simulink model "PID_nonlinear_improved_practical"  (R2022b)
settings: Solver=VariableStepAuto  StartTime=0.0  StopTime=20  RelTol=1e-3
values from neighbouring files (symbols this model uses):
  bias_acc = rand*0.05-0.025    [config.m]
  bias_gyro = rand*10-5    [config.m]
  f = 0.035    [config.m]
  g = 9.8    [config.m]
  Jx = 2*Mc*R^2/5 + 2*m*l^2    (= 0.0448)    [config.m]
  Jy = 2*Mc*R^2/5 + 2*m*l^2    (= 0.0448)    [config.m]
  Jz = 2*Mc*R^2/5 + 4*m*l^2    (= 0.0808)    [config.m]
  Kd_pitch = 15    [config.m]
  Kd_roll = 15    [config.m]
  Kd_yaw = 15    [config.m]
  Kd_z = 15    [config.m]
  Ki_pitch = 1    [config.m]
  Ki_roll = 1    [config.m]
  Ki_yaw = 1    [config.m]
  Ki_z = 10    [config.m]
  Kp_pitch = 80    [config.m]
  Kp_roll = 80    [config.m]
  Kp_yaw = 80    [config.m]
  Kp_z = 80    [config.m]
  M = Mc + 4*m    (= 3)    [config.m]
  S = 0.6231    [config.m]
  Wind_phi = 0    [config.m]
  Wind_theta = 0    [config.m]
  WorkTemperature = 30    [config.m]
libraries: simulink x2
settings Model: Creator=cxk  LastModifiedBy=cxk

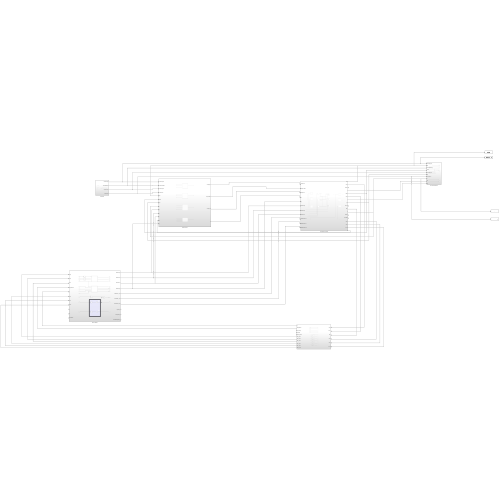
[thumbnail: Simulink's stored preview of the top-level diagram]
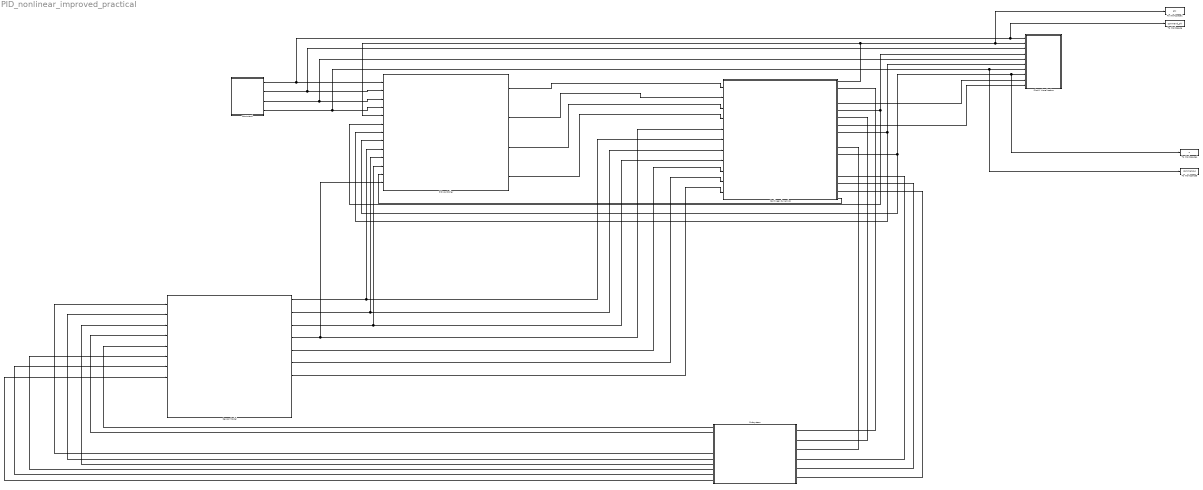
== system PID_nonlinear_improved_practical ==
  Command : Subsystem
  Nonlinear dynamics : Subsystem
  PID controller : Subsystem
  Plot & Visualization : Subsystem
  Sensor Model : Subsystem
  Subsystem : Subsystem
  To Workspace : ToWorkspace  VariableName=command_phi  SaveFormat=Timeseries  SampleTime=-1
  To Workspace1 : ToWorkspace  VariableName=phi  SaveFormat=Timeseries  SampleTime=-1
  To Workspace4 : ToWorkspace  VariableName=z  SaveFormat=Timeseries  SampleTime=-1
  To Workspace5 : ToWorkspace  VariableName=command_z  SaveFormat=Timeseries  SampleTime=-1
  wires:
  Nonlinear dynamics/8(psi) -> PID controller/7(psi), Plot & Visualization/6(psi)
  Nonlinear dynamics/5(theta) -> PID controller/6(theta), Plot & Visualization/4(theta)
  PID controller/4(F) -> Nonlinear dynamics/4(F)
  PID controller/1(Torque phi) -> Nonlinear dynamics/1(Torque Phi)
  PID controller/2(Torque theta) -> Nonlinear dynamics/2(Torque Theta)
  PID controller/3(Torque psi) -> Nonlinear dynamics/3(Torque Psi)
  Command/3(command psi) -> PID controller/3("command psi "), Plot & Visualization/5(command psi)
  Command/2(command theta) -> PID controller/2(command theta), Plot & Visualization/3(command theta)
  Nonlinear dynamics/4(x) -> Plot & Visualization/9(pn)
  Nonlinear dynamics/7(y) -> Plot & Visualization/10(pe)
  Subsystem/1(g) -> Sensor Model/5(g)
  Subsystem/2(temperature) -> Sensor Model/4(Temperature)
  Sensor Model/4(Measured g) -> Nonlinear dynamics/5(g), PID controller/13(g)
  Subsystem/6(dot p_real) -> Sensor Model/1(dot p)
  Subsystem/7(dot q_real) -> Sensor Model/2(dot q)
  Subsystem/8(dot r_real) -> Sensor Model/3(dot r)
  Subsystem/9(dot u_real) -> Sensor Model/6(dot u)
  Subsystem/10(dot v_real) -> Sensor Model/7(dot v)
  Subsystem/11(dot w_real) -> Sensor Model/8(dot w)
  Sensor Model/1(Measured p) -> Nonlinear dynamics/6(measured p), PID controller/9(p)
  Sensor Model/2(Measured q) -> Nonlinear dynamics/7(measured q), PID controller/10(q)
  Sensor Model/3(Measured r) -> Nonlinear dynamics/8(measured r), PID controller/11(r)
  Nonlinear dynamics/2(dot p) -> Subsystem/1(dot p)
  Nonlinear dynamics/6(dot q) -> Subsystem/2("dot q ")
  Nonlinear dynamics/10(dot r) -> Subsystem/3(dot r)
  Nonlinear dynamics/14(dot u) -> Subsystem/4(dot u)
  Nonlinear dynamics/15(dot v) -> Subsystem/5(dot v)
  Nonlinear dynamics/16(dot w) -> Subsystem/6(dot w)
  Sensor Model/5(Measured u_dot) -> Nonlinear dynamics/9(measured dot u)
  Sensor Model/6(Measured v_dot) -> Nonlinear dynamics/10(measured dot v)
  Sensor Model/7(Measured w_dot) -> Nonlinear dynamics/11(measured dot w)
  Nonlinear dynamics/17(w) -> PID controller/12(w)
  Nonlinear dynamics/11(z) -> PID controller/8(z), To Workspace4/1, Plot & Visualization/8(z)
  Nonlinear dynamics/1(Phi) -> To Workspace1/1, Plot & Visualization/2(phi), PID controller/5(phi)
  Command/4(command z) -> To Workspace5/1, Plot & Visualization/7(command z), PID controller/4(command z)
  Command/1(command phi) -> PID controller/1(command phi), To Workspace/1, Plot & Visualization/1(command phi)

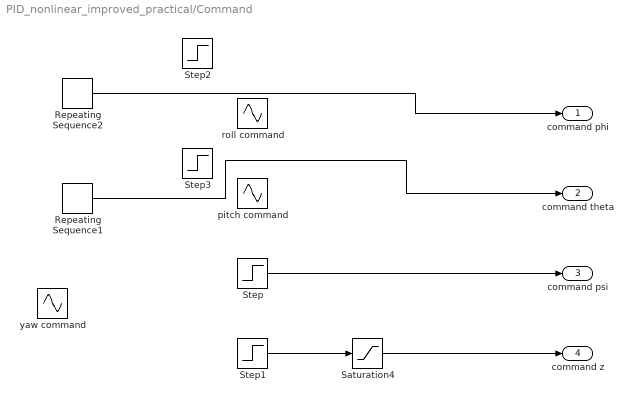
== system PID_nonlinear_improved_practical/Command ==
  Repeating Sequence1 : simulink/Sources/Repeating Sequence  rep_seq_t="[0 1 1.01  3 3.01 4 4.01 6]"  rep_seq_y=[0 0 0.68 0.68 -0.68 -0.68 0 0 ]
  Repeating Sequence2 : simulink/Sources/Repeating Sequence  rep_seq_t="[0 2 2.01  4 4.01 5 5.01 6]"  rep_seq_y=[0 0 0.68 0.68 -0.68 -0.68 0 0 ]
  Saturation4 : Saturate  UpperLimit=5  LowerLimit=-5
  Step : Step  Time=3  After=pi/4  SampleTime=0
  Step1 : Step  Time=2  After=-3  SampleTime=0
  Step2 : Step  Time=3  After=0.68  SampleTime=0
  Step3 : Step  Time=3  After=0.68  SampleTime=0
  pitch command : Sin  Amplitude=0.68  Frequency=0.5  SampleTime=0
  roll command : Sin  Amplitude=0.68  Frequency=0.5  SampleTime=0
  yaw command : Sin  Amplitude=pi  Frequency=0.5  SampleTime=0
  command phi : Outport
  command theta : Outport  Port=2
  command psi : Outport  Port=3
  command z : Outport  Port=4
  wires:
  Step1/1 -> Saturation4/1
  Saturation4/1 -> command z/1
  Step/1 -> command psi/1
  Repeating Sequence2/1 -> command phi/1
  Repeating Sequence1/1 -> command theta/1

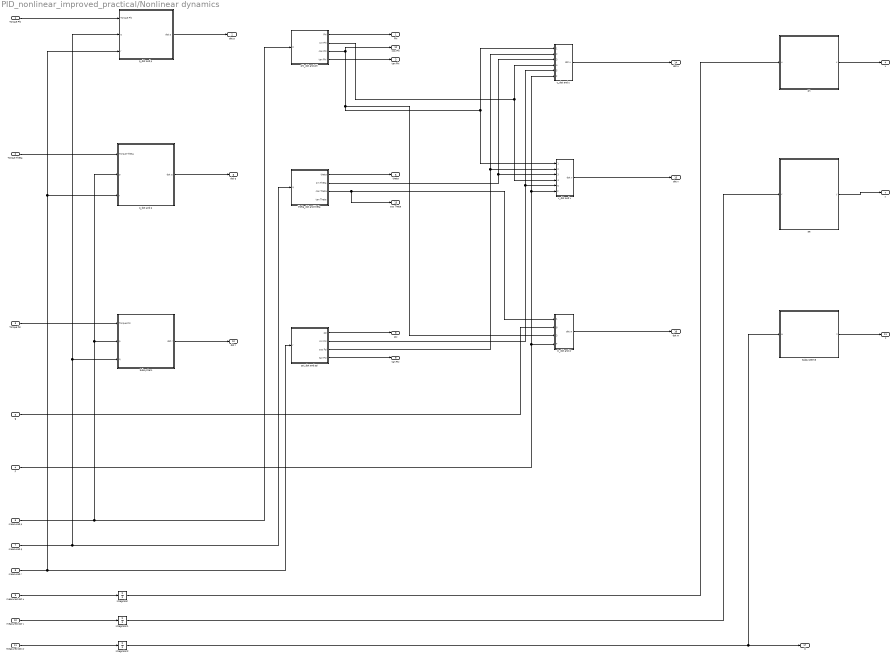
== system PID_nonlinear_improved_practical/Nonlinear dynamics ==
  Torque Phi : Inport
  Torque Theta : Inport  Port=2
  Torque Psi : Inport  Port=3
  F : Inport  Port=4
  g : Inport  Port=5
  measured p : Inport  Port=6
  measured q : Inport  Port=7
  measured r : Inport  Port=8
  measured dot u : Inport  Port=9
  measured dot v : Inport  Port=10
  measured dot w : Inport  Port=11
  Integrator : Integrator
  Integrator1 : Integrator
  Integrator2 : Integrator
  Subsystem : Subsystem
  Subsystem3 : Subsystem
  p_dot and p : Subsystem
  pe : Subsystem
  phi_dot and phi : Subsystem
  pn : Subsystem
  psi_dot and psi : Subsystem
  q_dot and q : Subsystem
  theta_dot and theta : Subsystem
  u_dot and u : Subsystem
  v_dot and v : Subsystem
  w_dot and w : Subsystem
  Phi : Outport
  dot p : Outport  Port=2
  tan Phi : Outport  Port=3
  x : Outport  Port=4
  theta : Outport  Port=5
  dot q : Outport  Port=6
  y : Outport  Port=7
  psi : Outport  Port=8
  tan Psi : Outport  Port=9
  dot r : Outport  Port=10
  z : Outport  Port=11
  cos Phi : Outport  Port=12
  cos Theta : Outport  Port=13
  dot u : Outport  Port=14
  dot v : Outport  Port=15
  dot w : Outport  Port=16
  w : Outport  Port=17
  wires:
  p_dot and p/1(dot p) -> dot p/1
  pe/1(y) -> y/1
  Torque Psi/1 -> Subsystem/1(Torque Psi)
  theta_dot and theta/1(theta) -> theta/1
  phi_dot and phi/1(Phi) -> Phi/1
  measured p/1 -> phi_dot and phi/1(p), Subsystem/2(p), q_dot and q/2(p)
  g/1 -> w_dot and w/2(g)
  phi_dot and phi/3(cos Phi) -> cos Phi/1, v_dot and v/1(cos phi), u_dot and u/1(cos phi), w_dot and w/3(cos phi)
  psi_dot and psi/3(cos Psi) -> u_dot and u/2(cos psi), v_dot and v/2(cos psi)
  psi_dot and psi/2(sin Psi) -> v_dot and v/5(sin psi), u_dot and u/5(sin psi)
  measured r/1 -> psi_dot and psi/1(r), p_dot and p/3(r), q_dot and q/3(r)
  theta_dot and theta/3(cos Theta) -> cos Theta/1, w_dot and w/1(cos theta)
  F/1 -> w_dot and w/4(F), v_dot and v/6(F), u_dot and u/6(F)
  Subsystem3/1(z) -> z/1
  measured q/1 -> theta_dot and theta/1(q), Subsystem/3(q), p_dot and p/2(q)
  psi_dot and psi/4(tan Psi) -> tan Psi/1
  q_dot and q/1(dot q) -> dot q/1
  Integrator1/1 -> pe/1(v)
  Subsystem/1(dot r) -> dot r/1
  measured dot w/1 -> Integrator2/1
  Integrator/1 -> pn/1(u)
  Integrator2/1 -> w/1, Subsystem3/1(w)
  phi_dot and phi/2(sin Phi) -> v_dot and v/4(sin phi), u_dot and u/4(sin phi)
  phi_dot and phi/4(tan Phi) -> tan Phi/1
  Torque Phi/1 -> p_dot and p/1(Torque Phi)
  theta_dot and theta/2(sin Theta) -> v_dot and v/3(sin theta), u_dot and u/3(sin theta)
  w_dot and w/1(dot w) -> dot w/1
  measured dot v/1 -> Integrator1/1
  pn/1(x) -> x/1
  psi_dot and psi/1(psi) -> psi/1
  u_dot and u/1(dot u) -> dot u/1
  v_dot and v/1(dot v) -> dot v/1
  measured dot u/1 -> Integrator/1
  Torque Theta/1 -> q_dot and q/1(Torque Theta)

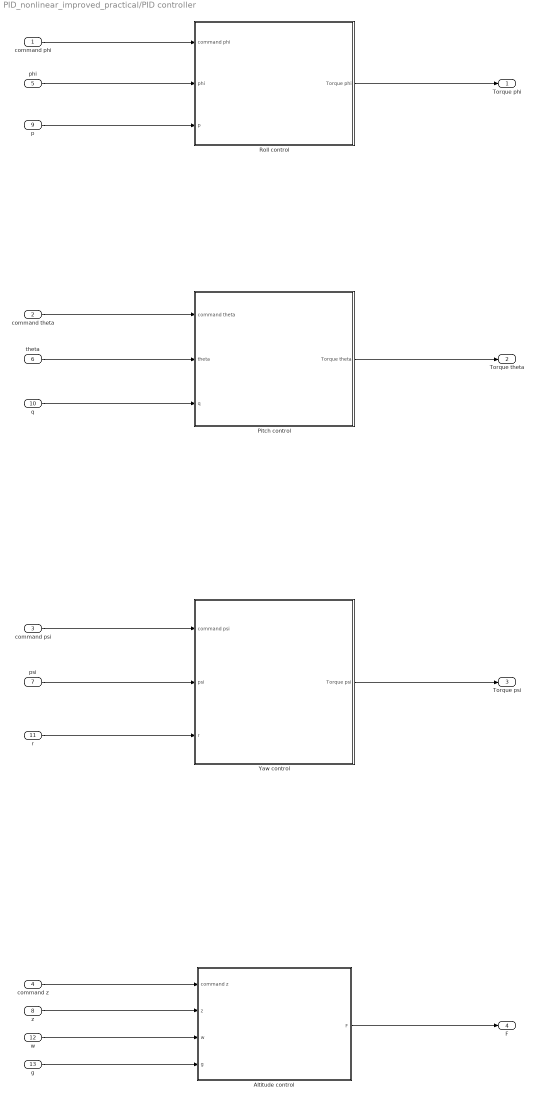
== system PID_nonlinear_improved_practical/PID controller ==
  command phi : Inport
  command theta : Inport  Port=2
  "command psi " : Inport  Port=3
  command z : Inport  Port=4
  phi : Inport  Port=5
  theta : Inport  Port=6
  psi : Inport  Port=7
  z : Inport  Port=8
  p : Inport  Port=9
  q : Inport  Port=10
  r : Inport  Port=11
  w : Inport  Port=12
  g : Inport  Port=13
  Altitude control : Subsystem
  Pitch control : Subsystem
  Roll control : Subsystem
  Yaw control : Subsystem
  Torque phi : Outport
  Torque theta : Outport  Port=2
  Torque psi : Outport  Port=3
  F : Outport  Port=4
  wires:
  phi/1 -> Roll control/2(phi)
  command phi/1 -> Roll control/1(command phi)
  theta/1 -> Pitch control/2(theta)
  command theta/1 -> Pitch control/1(command theta)
  command z/1 -> Altitude control/1(command z)
  Yaw control/1(Torque psi) -> Torque psi/1
  z/1 -> Altitude control/2(z)
  "command psi "/1 -> Yaw control/1("command psi ")
  w/1 -> Altitude control/3(w)
  q/1 -> Pitch control/3(q)
  Altitude control/1(F) -> F/1
  Pitch control/1(Torque theta) -> Torque theta/1
  psi/1 -> Yaw control/2(psi)
  Roll control/1(Torque phi) -> Torque phi/1
  r/1 -> Yaw control/3(r)
  p/1 -> Roll control/3(p)
  g/1 -> Altitude control/4(g)

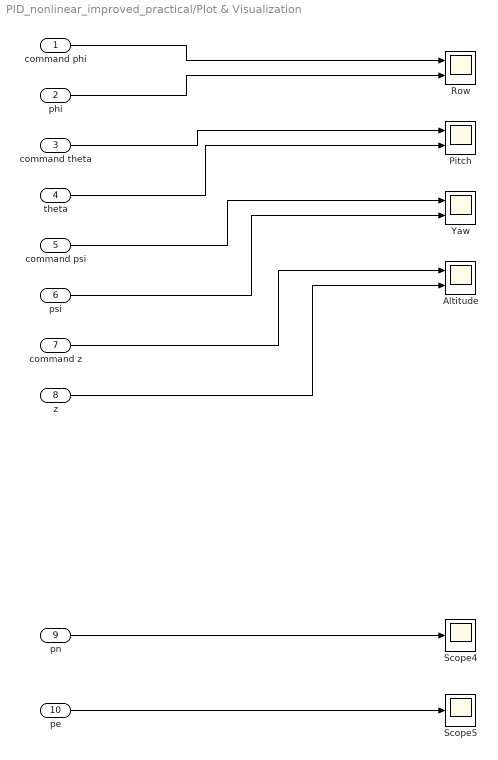
== system PID_nonlinear_improved_practical/Plot & Visualization ==
  command phi : Inport
  phi : Inport  Port=2
  command theta : Inport  Port=3
  theta : Inport  Port=4
  command psi : Inport  Port=5
  psi : Inport  Port=6
  command z : Inport  Port=7
  z : Inport  Port=8
  pn : Inport  Port=9
  pe : Inport  Port=10
  Altitude : Scope  NumInputPorts=2
  Pitch : Scope  NumInputPorts=2
  Row : Scope  NumInputPorts=2
  Scope4 : Scope
  Scope5 : Scope
  Yaw : Scope  NumInputPorts=2
  wires:
  z/1 -> Altitude/2
  command phi/1 -> Row/1
  phi/1 -> Row/2
  command z/1 -> Altitude/1
  command psi/1 -> Yaw/1
  pe/1 -> Scope5/1
  psi/1 -> Yaw/2
  pn/1 -> Scope4/1
  theta/1 -> Pitch/2
  command theta/1 -> Pitch/1

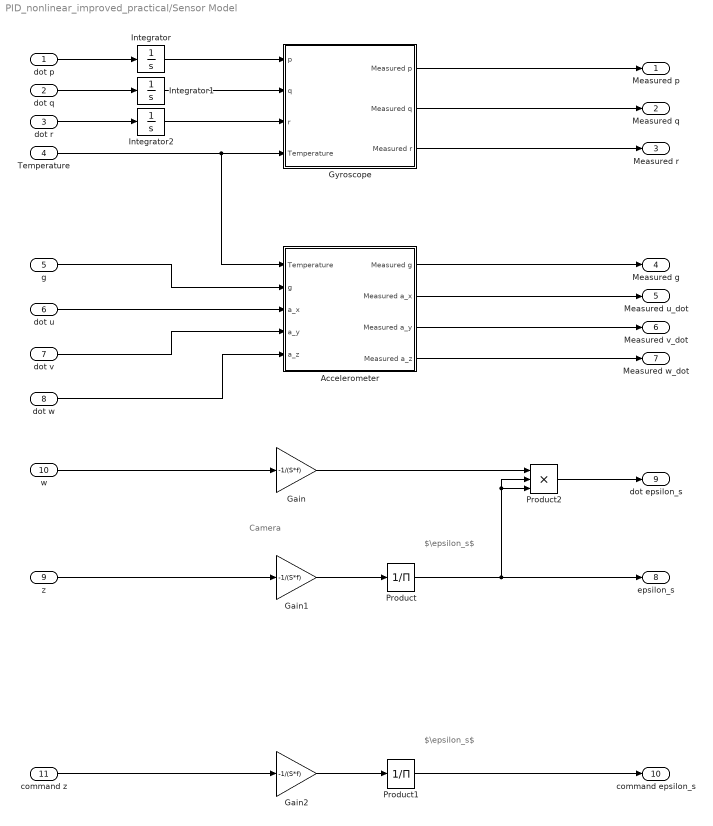
== system PID_nonlinear_improved_practical/Sensor Model ==
  note: Camera
  note: $\epsilon_s$
  note: $\epsilon_s$
  dot p : Inport
  dot q : Inport  Port=2
  dot r : Inport  Port=3
  Temperature : Inport  Port=4
  g : Inport  Port=5
  dot u : Inport  Port=6
  dot v : Inport  Port=7
  dot w : Inport  Port=8
  z : Inport  Port=9
  w : Inport  Port=10
  command z : Inport  Port=11
  Accelerometer : Subsystem
  Gain : Gain  Gain=-1/(S*f)
  Gain1 : Gain  Gain=-1/(S*f)
  Gain2 : Gain  Gain=-1/(S*f)
  Gyroscope : Subsystem
  Integrator : Integrator
  Integrator1 : Integrator
  Integrator2 : Integrator
  Product : Product  Inputs=/
  Product1 : Product  Inputs=/
  Product2 : Product  Inputs=3
  Measured p : Outport
  Measured q : Outport  Port=2
  Measured r : Outport  Port=3
  Measured g : Outport  Port=4
  Measured u_dot : Outport  Port=5
  Measured v_dot : Outport  Port=6
  Measured w_dot : Outport  Port=7
  epsilon_s : Outport  Port=8
  dot epsilon_s : Outport  Port=9
  command epsilon_s : Outport  Port=10
  wires:
  dot p/1 -> Integrator/1
  dot q/1 -> Integrator1/1
  dot r/1 -> Integrator2/1
  Temperature/1 -> Accelerometer/1(Temperature), Gyroscope/4(Temperature)
  Gyroscope/1(Measured p) -> Measured p/1
  Gyroscope/2(Measured q) -> Measured q/1
  Gyroscope/3(Measured r) -> Measured r/1
  g/1 -> Accelerometer/2(g)
  dot u/1 -> Accelerometer/3(a_x)
  dot v/1 -> Accelerometer/4(a_y)
  dot w/1 -> Accelerometer/5(a_z)
  Accelerometer/1(Measured g) -> Measured g/1
  Accelerometer/2(Measured a_x) -> Measured u_dot/1
  Accelerometer/3(Measured a_y) -> Measured v_dot/1
  Accelerometer/4(Measured a_z) -> Measured w_dot/1
  z/1 -> Gain1/1
  Gain1/1 -> Product/1
  Product/1 -> Product2/3, Product2/2, epsilon_s/1
  Product1/1 -> command epsilon_s/1
  Gain2/1 -> Product1/1
  command z/1 -> Gain2/1
  w/1 -> Gain/1
  Gain/1 -> Product2/1
  Product2/1 -> dot epsilon_s/1
  Integrator/1 -> Gyroscope/1(p)
  Integrator1/1 -> Gyroscope/2(q)
  Integrator2/1 -> Gyroscope/3(r)

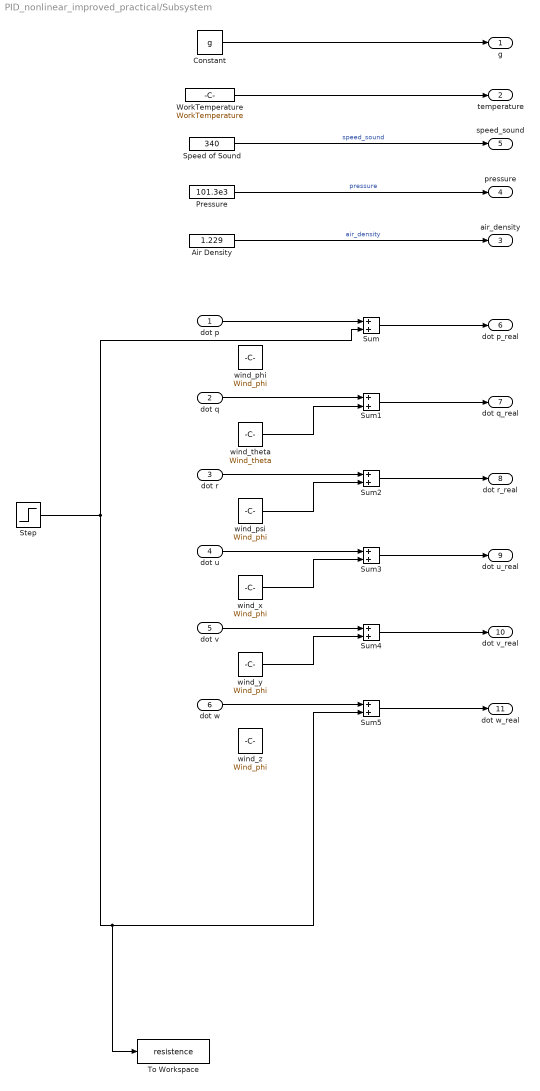
== system PID_nonlinear_improved_practical/Subsystem ==
  dot p : Inport
  "dot q " : Inport  Port=2
  dot r : Inport  Port=3
  dot u : Inport  Port=4
  dot v : Inport  Port=5
  dot w : Inport  Port=6
  Air Density : Constant  Value=1.229
  Constant : Constant  Value=g
  Pressure : Constant  Value=101.3e3
  Speed of Sound : Constant  Value=340
  Step : Step  Time=10  After=5  SampleTime=0
  Sum{,1..5} (6 alike) : Sum
  To Workspace : ToWorkspace  VariableName=resistence  SaveFormat=Timeseries  SampleTime=-1
  WorkTemperature : Constant  Value=WorkTemperature
  wind_phi : Constant  Value=Wind_phi
  wind_psi : Constant  Value=Wind_phi
  wind_theta : Constant  Value=Wind_theta
  wind_x : Constant  Value=Wind_phi
  wind_y : Constant  Value=Wind_phi
  wind_z : Constant  Value=Wind_phi
  g : Outport
  temperature : Outport  Port=2
  air_density : Outport  Port=3
  pressure : Outport  Port=4
  speed_sound : Outport  Port=5
  dot p_real : Outport  Port=6
  dot q_real : Outport  Port=7
  dot r_real : Outport  Port=8
  dot u_real : Outport  Port=9
  dot v_real : Outport  Port=10
  dot w_real : Outport  Port=11
  wires:
  Constant/1 -> g/1
  Air Density/1 -> air_density/1  "air_density"
  Speed of Sound/1 -> speed_sound/1  "speed_sound"
  WorkTemperature/1 -> temperature/1
  Pressure/1 -> pressure/1  "pressure"
  dot p/1 -> Sum/1
  Sum/1 -> dot p_real/1
  wind_theta/1 -> Sum1/2
  Sum1/1 -> dot q_real/1
  "dot q "/1 -> Sum1/1
  wind_psi/1 -> Sum2/2
  Sum2/1 -> dot r_real/1
  dot r/1 -> Sum2/1
  wind_x/1 -> Sum3/2
  Sum3/1 -> dot u_real/1
  dot u/1 -> Sum3/1
  wind_y/1 -> Sum4/2
  Sum4/1 -> dot v_real/1
  dot v/1 -> Sum4/1
  Sum5/1 -> dot w_real/1
  dot w/1 -> Sum5/1
  Step/1 -> Sum/2, Sum5/2, To Workspace/1

== system PID_nonlinear_improved_practical/Nonlinear dynamics/Subsystem ==
  note: $\dot r$
  note: ${(J_x-J_y) \over J_z}pq$
  note: r_dot and r
  note: $r$
  Torque Psi : Inport
  p : Inport  Port=2
  q : Inport  Port=3
  Gain2 : Gain  Gain=1/Jz
  Gain20 : Gain  Gain=(Jx-Jy)/Jz
  Product2 : Product
  Sum11 : Sum
  dot r : Outport
  wires:
  Gain20/1 -> Product2/1
  Torque Psi/1 -> Gain2/1
  p/1 -> Gain20/1
  Product2/1 -> Sum11/2
  q/1 -> Product2/2
  Sum11/1 -> dot r/1
  Gain2/1 -> Sum11/1

== system PID_nonlinear_improved_practical/Nonlinear dynamics/Subsystem3 ==
  note: $h$
  note: $\dot h$
  w : Inport
  Integrator : Integrator
  z : Outport
  wires:
  w/1 -> Integrator/1
  Integrator/1 -> z/1

== system PID_nonlinear_improved_practical/Nonlinear dynamics/p_dot and p ==
  note: p_dot and p
  note: ${(J_y-J_z) \over J_x}qr$
  note: $\dot p$
  note: $p$
  Torque Phi : Inport
  q : Inport  Port=2
  r : Inport  Port=3
  Gain12 : Gain  Gain=1/Jx
  Gain17 : Gain  Gain=(Jy-Jz)/Jx
  Product : Product
  Sum9 : Sum
  dot p : Outport
  wires:
  Product/1 -> Sum9/2
  r/1 -> Product/2
  Sum9/1 -> dot p/1
  Gain17/1 -> Product/1
  Gain12/1 -> Sum9/1
  Torque Phi/1 -> Gain12/1
  q/1 -> Gain17/1

== system PID_nonlinear_improved_practical/Nonlinear dynamics/pe ==
  note: $\dot p_e$
  note: $p_e$
  v : Inport
  Integrator : Integrator
  y : Outport
  wires:
  v/1 -> Integrator/1
  Integrator/1 -> y/1

== system PID_nonlinear_improved_practical/Nonlinear dynamics/phi_dot and phi ==
  note: $\phi$
  note: $\dot \phi$
  p : Inport
  Integrator1 : Integrator
  Subsystem1 : Subsystem
  Phi : Outport
  sin Phi : Outport  Port=2
  cos Phi : Outport  Port=3
  tan Phi : Outport  Port=4
  wires:
  Subsystem1/2(cos Phi) -> cos Phi/1
  Subsystem1/1(sin Phi) -> sin Phi/1
  Integrator1/1 -> Phi/1, Subsystem1/1(phi)
  p/1 -> Integrator1/1
  Subsystem1/3(tan Phi) -> tan Phi/1

== system PID_nonlinear_improved_practical/Nonlinear dynamics/pn ==
  note: $\dot p_n$
  note: $p_n$
  u : Inport
  Integrator : Integrator
  x : Outport
  wires:
  u/1 -> Integrator/1
  Integrator/1 -> x/1

== system PID_nonlinear_improved_practical/Nonlinear dynamics/psi_dot and psi ==
  note: $\Psi$
  note: $\dot \Psi$
  r : Inport
  Integrator4 : Integrator
  Subsystem2 : Subsystem
  psi : Outport
  sin Psi : Outport  Port=2
  cos Psi : Outport  Port=3
  tan Psi : Outport  Port=4
  wires:
  Subsystem2/2(cos Psi) -> cos Psi/1
  r/1 -> Integrator4/1
  Integrator4/1 -> psi/1, Subsystem2/1(psi)
  Subsystem2/1(sin Psi) -> sin Psi/1
  Subsystem2/3(tan Psi) -> tan Psi/1

== system PID_nonlinear_improved_practical/Nonlinear dynamics/q_dot and q ==
  note: $\dot q$
  note: ${(J_z-J_x) \over J_y}pr$
  note: q_dot and q
  note: $q$
  Torque Theta : Inport
  p : Inport  Port=2
  r : Inport  Port=3
  Gain16 : Gain  Gain=1/Jy
  Gain19 : Gain  Gain=(Jz-Jx)/Jy
  Product1 : Product
  Sum10 : Sum
  dot q : Outport
  wires:
  Gain16/1 -> Sum10/1
  Sum10/1 -> dot q/1
  r/1 -> Product1/2
  Gain19/1 -> Product1/1
  Product1/1 -> Sum10/2
  Torque Theta/1 -> Gain16/1
  p/1 -> Gain19/1

== system PID_nonlinear_improved_practical/Nonlinear dynamics/theta_dot and theta ==
  note: $\theta$
  note: $\dot \theta$
  q : Inport
  Integrator2 : Integrator
  Subsystem2 : Subsystem
  theta : Outport
  sin Theta : Outport  Port=2
  cos Theta : Outport  Port=3
  tan Theta : Outport  Port=4
  wires:
  Subsystem2/1(sin Theta) -> sin Theta/1
  q/1 -> Integrator2/1
  Integrator2/1 -> theta/1, Subsystem2/1(theta)
  Subsystem2/3(tan Theta) -> tan Theta/1
  Subsystem2/2(cos Theta) -> cos Theta/1

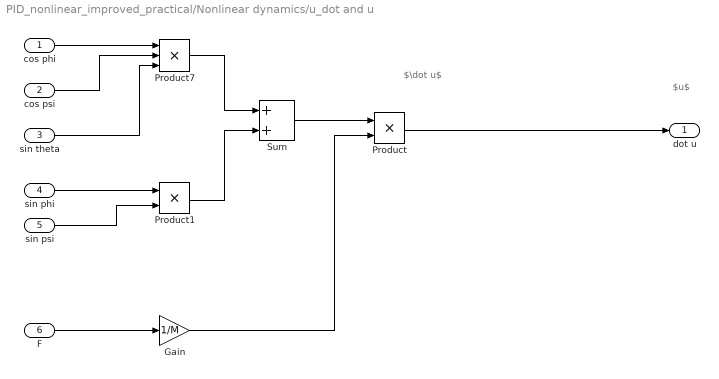
== system PID_nonlinear_improved_practical/Nonlinear dynamics/u_dot and u ==
  note: $\dot u$
  note: $u$
  cos phi : Inport
  cos psi : Inport  Port=2
  sin theta : Inport  Port=3
  sin phi : Inport  Port=4
  sin psi : Inport  Port=5
  F : Inport  Port=6
  Gain : Gain  Gain=1/M
  Product : Product
  Product1 : Product
  Product7 : Product  Inputs=3
  Sum : Sum
  dot u : Outport
  wires:
  Sum/1 -> Product/1
  Gain/1 -> Product/2
  Product7/1 -> Sum/1
  sin theta/1 -> Product7/3
  cos phi/1 -> Product7/1
  Product1/1 -> Sum/2
  F/1 -> Gain/1
  sin phi/1 -> Product1/1
  cos psi/1 -> Product7/2
  sin psi/1 -> Product1/2
  Product/1 -> dot u/1

== system PID_nonlinear_improved_practical/Nonlinear dynamics/v_dot and v ==
  note: $\dot v$
  note: $v$
  cos phi : Inport
  cos psi : Inport  Port=2
  sin theta : Inport  Port=3
  sin phi : Inport  Port=4
  sin psi : Inport  Port=5
  F : Inport  Port=6
  Gain : Gain  Gain=1/M
  Product : Product
  Product1 : Product
  Product7 : Product  Inputs=3
  Sum : Sum  Inputs=+-
  dot v : Outport
  wires:
  cos phi/1 -> Product7/1
  Product/1 -> dot v/1
  cos psi/1 -> Product7/2
  sin theta/1 -> Product7/3
  Sum/1 -> Product/1
  sin phi/1 -> Product1/1
  sin psi/1 -> Product1/2
  F/1 -> Gain/1
  Gain/1 -> Product/2
  Product7/1 -> Sum/1
  Product1/1 -> Sum/2

== system PID_nonlinear_improved_practical/Nonlinear dynamics/w_dot and w ==
  note: $\dot w$
  note: $w$
  cos theta : Inport
  g : Inport  Port=2
  cos phi : Inport  Port=3
  F : Inport  Port=4
  Gain : Gain  Gain=1/M
  Product8 : Product  Inputs=3
  Sum11 : Sum  Inputs=-+
  dot w : Outport
  wires:
  cos phi/1 -> Product8/3
  Product8/1 -> Sum11/2
  Sum11/1 -> dot w/1
  g/1 -> Sum11/1
  cos theta/1 -> Product8/1
  F/1 -> Gain/1
  Gain/1 -> Product8/2

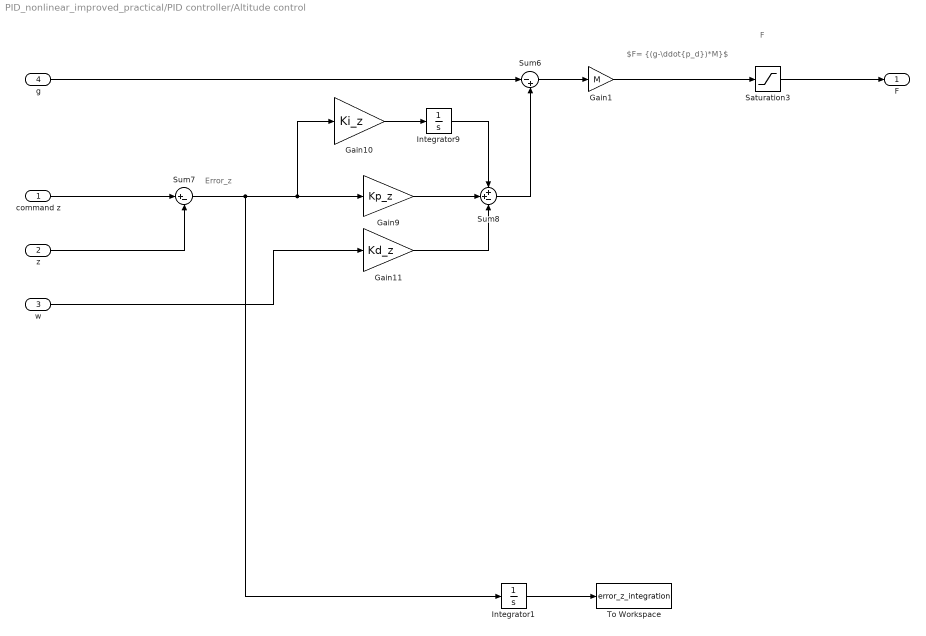
== system PID_nonlinear_improved_practical/PID controller/Altitude control ==
  note: $F= {(g-\ddot{p_d})*M}$
  note: Error_z
  note: F
  command z : Inport
  z : Inport  Port=2
  w : Inport  Port=3
  g : Inport  Port=4
  Gain1 : Gain  Gain=M
  Gain10 : Gain  Gain=Ki_z
  Gain11 : Gain  Gain=Kd_z
  Gain9 : Gain  Gain=Kp_z
  Integrator1 : Integrator
  Integrator9 : Integrator
  Saturation3 : Saturate  UpperLimit=g*M*10  LowerLimit=-2.97*M*10
  Sum6 : Sum  Inputs=|-+
  Sum7 : Sum  Inputs=|+-
  Sum8 : Sum  Inputs=++-
  To Workspace : ToWorkspace  VariableName=error_z_integration  SaveFormat=Timeseries  SampleTime=-1
  F : Outport
  wires:
  Sum6/1 -> Gain1/1
  Gain9/1 -> Sum8/2
  Integrator9/1 -> Sum8/1
  g/1 -> Sum6/1
  Gain10/1 -> Integrator9/1
  Sum8/1 -> Sum6/2
  Gain1/1 -> Saturation3/1
  command z/1 -> Sum7/1
  Gain11/1 -> Sum8/3
  Saturation3/1 -> F/1
  z/1 -> Sum7/2
  w/1 -> Gain11/1
  Integrator1/1 -> To Workspace/1
  Sum7/1 -> Gain10/1, Gain9/1, Integrator1/1

== system PID_nonlinear_improved_practical/PID controller/Pitch control ==
  note: $E_\theta=\theta_d-\theta$
  note: $\tau_\theta$
  command theta : Inport
  theta : Inport  Port=2
  q : Inport  Port=3
  Gain13 : Gain  Gain=Kp_pitch
  Gain14 : Gain  Gain=Ki_pitch
  Gain15 : Gain  Gain=Kd_pitch
  Integrator3 : Integrator
  Saturation1 : Saturate  UpperLimit=100  LowerLimit=-100
  Sum2 : Sum  Inputs=|+-
  Sum3 : Sum  Inputs=++-
  Torque theta : Outport
  wires:
  command theta/1 -> Sum2/1
  Sum2/1 -> Gain14/1, Gain13/1
  Gain14/1 -> Integrator3/1
  Sum3/1 -> Saturation1/1
  Integrator3/1 -> Sum3/1
  Gain15/1 -> Sum3/3
  theta/1 -> Sum2/2
  Gain13/1 -> Sum3/2
  Saturation1/1 -> Torque theta/1
  q/1 -> Gain15/1

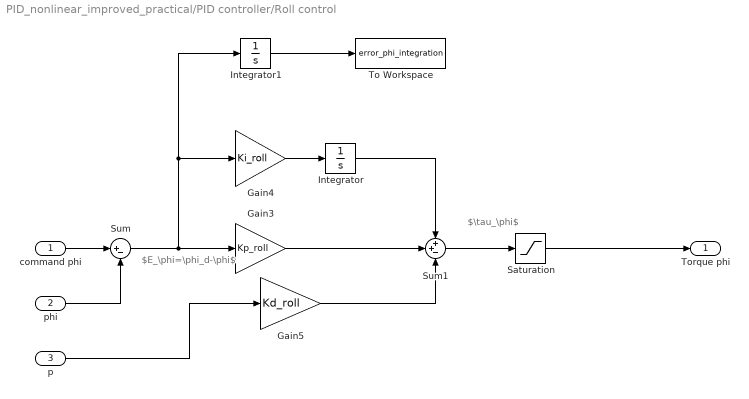
== system PID_nonlinear_improved_practical/PID controller/Roll control ==
  note: $\tau_\phi$
  note: $E_\phi=\phi_d-\phi$
  command phi : Inport
  phi : Inport  Port=2
  p : Inport  Port=3
  Gain3 : Gain  Gain=Kp_roll
  Gain4 : Gain  Gain=Ki_roll
  Gain5 : Gain  Gain=Kd_roll
  Integrator : Integrator
  Integrator1 : Integrator
  Saturation : Saturate  UpperLimit=100  LowerLimit=-100
  Sum : Sum  Inputs=|+-
  Sum1 : Sum  Inputs=++-
  To Workspace : ToWorkspace  VariableName=error_phi_integration  SaveFormat=Timeseries  SampleTime=-1
  Torque phi : Outport
  wires:
  Integrator/1 -> Sum1/1
  Gain4/1 -> Integrator/1
  Gain5/1 -> Sum1/3
  Saturation/1 -> Torque phi/1
  Sum1/1 -> Saturation/1
  Gain3/1 -> Sum1/2
  command phi/1 -> Sum/1
  phi/1 -> Sum/2
  p/1 -> Gain5/1
  Sum/1 -> Integrator1/1, Gain4/1, Gain3/1
  Integrator1/1 -> To Workspace/1

== system PID_nonlinear_improved_practical/PID controller/Yaw control ==
  note: $E_\Psi=\Psi-\Psi_d$
  note: $\tau_\psi$
  "command psi " : Inport
  psi : Inport  Port=2
  r : Inport  Port=3
  Gain6 : Gain  Gain=Kd_yaw
  Gain7 : Gain  Gain=Kp_yaw
  Gain8 : Gain  Gain=Ki_yaw
  Integrator7 : Integrator
  Saturation2 : Saturate  UpperLimit=100  LowerLimit=-100
  Sum4 : Sum  Inputs=---
  Sum5 : Sum  Inputs=|-+
  Torque psi : Outport
  wires:
  Sum4/1 -> Saturation2/1
  Integrator7/1 -> Sum4/1
  Gain8/1 -> Integrator7/1
  psi/1 -> Sum5/2
  Sum5/1 -> Gain8/1, Gain7/1
  Gain7/1 -> Sum4/2
  Gain6/1 -> Sum4/3
  "command psi "/1 -> Sum5/1
  Saturation2/1 -> Torque psi/1
  r/1 -> Gain6/1

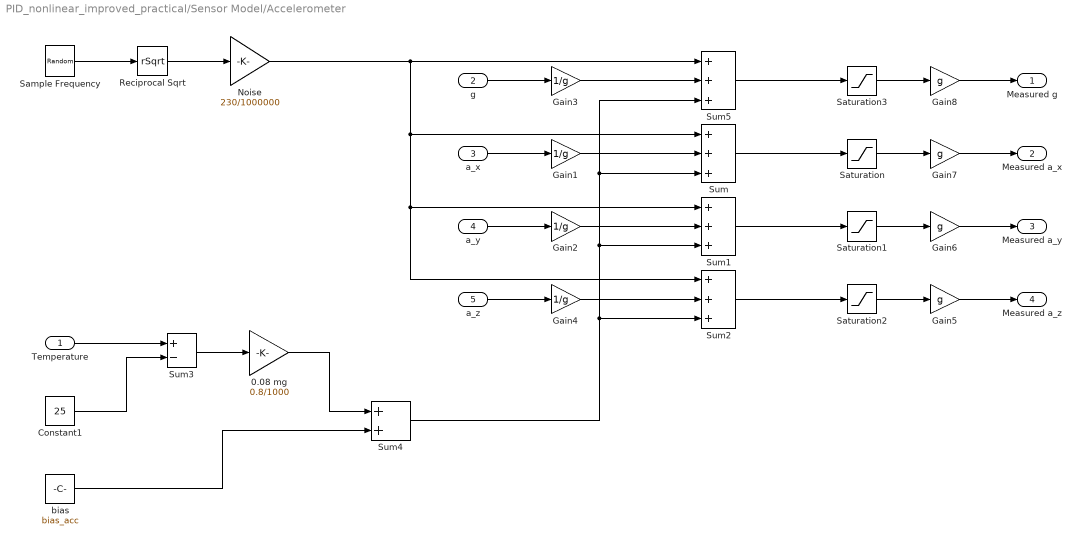
== system PID_nonlinear_improved_practical/Sensor Model/Accelerometer ==
  Temperature : Inport
  g : Inport  Port=2
  a_x : Inport  Port=3
  a_y : Inport  Port=4
  a_z : Inport  Port=5
  0.08 mg : Gain  Gain=0.8/1000
  Constant1 : Constant  Value=25
  Gain{1..4} (4 alike) : Gain  Gain=1/g
  Gain{5..8} (4 alike) : Gain  Gain=g
  Noise : Gain  Gain=230/1000000
  Reciprocal Sqrt : Sqrt  Operator=rSqrt
  Sample Frequency : UniformRandomNumber  Minimum=4.5  Maximum=1125  SampleTime=0.1
  Saturation{,1..3} (4 alike) : Saturate  UpperLimit=4  LowerLimit=-4
  Sum{,1..2,5} (4 alike) : Sum  Inputs=+++
  Sum3 : Sum  Inputs=+-
  Sum4 : Sum
  bias : Constant  Value=bias_acc
  Measured g : Outport
  Measured a_x : Outport  Port=2
  Measured a_y : Outport  Port=3
  Measured a_z : Outport  Port=4
  wires:
  Saturation1/1 -> Gain6/1
  Saturation/1 -> Gain7/1
  a_y/1 -> Gain2/1
  0.08 mg/1 -> Sum4/1
  Temperature/1 -> Sum3/1
  a_x/1 -> Gain1/1
  Sum2/1 -> Saturation2/1
  Saturation2/1 -> Gain5/1
  a_z/1 -> Gain4/1
  Sample Frequency/1 -> Reciprocal Sqrt/1
  Sum1/1 -> Saturation1/1
  bias/1 -> Sum4/2
  Constant1/1 -> Sum3/2
  Sum/1 -> Saturation/1
  Sum3/1 -> 0.08 mg/1
  Reciprocal Sqrt/1 -> Noise/1
  Sum5/1 -> Saturation3/1
  Sum4/1 -> Sum5/3, Sum/3, Sum1/3, Sum2/3
  Noise/1 -> Sum2/1, Sum1/1, Sum/1, Sum5/1
  Saturation3/1 -> Gain8/1
  g/1 -> Gain3/1
  Gain1/1 -> Sum/2
  Gain2/1 -> Sum1/2
  Gain3/1 -> Sum5/2
  Gain4/1 -> Sum2/2
  Gain5/1 -> Measured a_z/1
  Gain6/1 -> Measured a_y/1
  Gain7/1 -> Measured a_x/1
  Gain8/1 -> Measured g/1

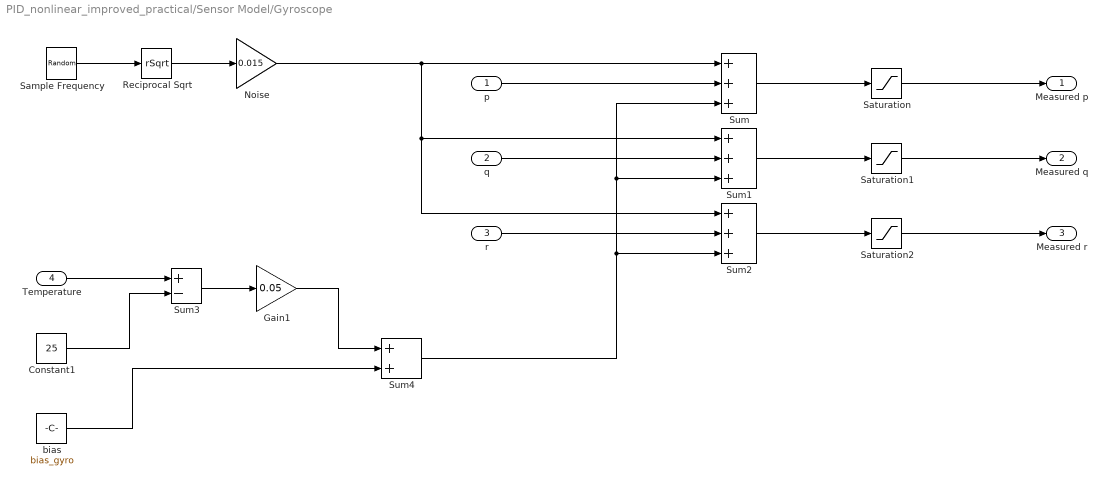
== system PID_nonlinear_improved_practical/Sensor Model/Gyroscope ==
  p : Inport
  q : Inport  Port=2
  r : Inport  Port=3
  Temperature : Inport  Port=4
  Constant1 : Constant  Value=25
  Gain1 : Gain  Gain=0.05
  Noise : Gain  Gain=0.015
  Reciprocal Sqrt : Sqrt  Operator=rSqrt
  Sample Frequency : UniformRandomNumber  Minimum=4.4  Maximum=1125  SampleTime=0.1
  Saturation : Saturate  UpperLimit=500  LowerLimit=-500
  Saturation1 : Saturate  UpperLimit=500  LowerLimit=-500
  Saturation2 : Saturate  UpperLimit=500  LowerLimit=-500
  Sum : Sum  Inputs=+++
  Sum1 : Sum  Inputs=+++
  Sum2 : Sum  Inputs=+++
  Sum3 : Sum  Inputs=+-
  Sum4 : Sum
  bias : Constant  Value=bias_gyro
  Measured p : Outport
  Measured q : Outport  Port=2
  Measured r : Outport  Port=3
  wires:
  Saturation1/1 -> Measured q/1
  Saturation/1 -> Measured p/1
  q/1 -> Sum1/2
  Sum4/1 -> Sum1/3, Sum/3, Sum2/3
  Noise/1 -> Sum2/1, Sum1/1, Sum/1
  Gain1/1 -> Sum4/1
  Temperature/1 -> Sum3/1
  p/1 -> Sum/2
  Sum2/1 -> Saturation2/1
  Saturation2/1 -> Measured r/1
  r/1 -> Sum2/2
  Sample Frequency/1 -> Reciprocal Sqrt/1
  Sum1/1 -> Saturation1/1
  bias/1 -> Sum4/2
  Constant1/1 -> Sum3/2
  Sum/1 -> Saturation/1
  Sum3/1 -> Gain1/1
  Reciprocal Sqrt/1 -> Noise/1

== system PID_nonlinear_improved_practical/Nonlinear dynamics/phi_dot and phi/Subsystem1 ==
  phi : Inport
  Trigonometric Function : Trigonometry
  Trigonometric Function1 : Trigonometry  Operator=cos
  Trigonometric Function2 : Trigonometry  Operator=tan
  sin Phi : Outport
  cos Phi : Outport  Port=2
  tan Phi : Outport  Port=3
  wires:
  phi/1 -> Trigonometric Function2/1, Trigonometric Function1/1, Trigonometric Function/1
  Trigonometric Function2/1 -> tan Phi/1
  Trigonometric Function/1 -> sin Phi/1
  Trigonometric Function1/1 -> cos Phi/1

== system PID_nonlinear_improved_practical/Nonlinear dynamics/psi_dot and psi/Subsystem2 ==
  psi : Inport
  Trigonometric Function : Trigonometry
  Trigonometric Function1 : Trigonometry  Operator=cos
  Trigonometric Function2 : Trigonometry  Operator=tan
  sin Psi : Outport
  cos Psi : Outport  Port=2
  tan Psi : Outport  Port=3
  wires:
  psi/1 -> Trigonometric Function2/1, Trigonometric Function1/1, Trigonometric Function/1
  Trigonometric Function2/1 -> tan Psi/1
  Trigonometric Function/1 -> sin Psi/1
  Trigonometric Function1/1 -> cos Psi/1

== system PID_nonlinear_improved_practical/Nonlinear dynamics/theta_dot and theta/Subsystem2 ==
  theta : Inport
  Trigonometric Function : Trigonometry
  Trigonometric Function1 : Trigonometry  Operator=cos
  Trigonometric Function2 : Trigonometry  Operator=tan
  sin Theta : Outport
  cos Theta : Outport  Port=2
  tan Theta : Outport  Port=3
  wires:
  theta/1 -> Trigonometric Function2/1, Trigonometric Function1/1, Trigonometric Function/1
  Trigonometric Function2/1 -> tan Theta/1
  Trigonometric Function/1 -> sin Theta/1
  Trigonometric Function1/1 -> cos Theta/1
